simulink library "siltestlib"  (R2015b)
settings: Solver=VariableStepAuto  SolverMode=SingleTasking  StartTime=0.0  StopTime=10.0  RelTol=1e-3
settings Model: ExtModeArmWhenConnect=off  Creator=13188  LastModifiedBy=13188
settings DataIOCC: SaveFormat=Array  SignalLoggingSaveFormat=ModelDataLogs
settings OptimizationCC: BlockReduction=off  BooleanDataType=off
settings DebuggingCC: SaveWithParameterizedLinksMsg=none  UnderspecifiedInitializationDetection=Classic  MergeDetectMultiDrivingBlocksExec=none  SignalResolutionControl=TryResolveAllWithWarning  MultiTaskDSMMsg=warning  MultiTaskCondExecSysMsg=none  StrictBusMsg=None
settings HardwareCC: ProdBitPerPointer=32  ProdLargestAtomicFloat=None  ProdIntDivRoundTo=Undefined  ProdEndianess=Unspecified  ProdWordSize=32  ProdHWDeviceType=32-bit Generic  TargetUnknown=on
settings RTWCC: MakeCommand=make_rti  RetainRTWFile=on
settings ConfigComp: CovModelRefEnable=Off

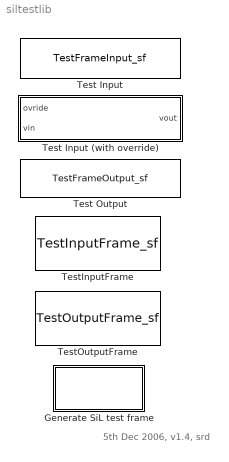
== system siltestlib ==
  note: 5th Dec 2006, v1.4, srd
  Generate SiL test frame : Subsystem  Description=Generate SiL\ntest frame  TreatAsAtomicUnit=on  mask(Generate SiL test frame button.){}
      mask help: Calls the function gen_sil_test_frame.
      settings: OpenFcn=|
      | if exist('gen_sil_test_frame','file'), gen_sil_test_frame(gcs); else,
      | fprintf('Error: gen_sil_test_frame is not on the matlab path.\n'); end
      mask Help: Calls the function gen_sil_test_frame.
      mask Display: fprintf('Generate SiL\ntest frame');
  Test Input : S-Function  FunctionName=TestFrameInput_sf  Parameters=varname,sampletime  SFunctionDeploymentMode=off  EnableBusSupport=off  mask(Test Input){varname=<UNDEFINED>, sampletime=-1}
      mask prompts: varname "Name:"; sampletime "Sample Time:"
      mask help: Outputs the value of a Test Input variable from an Excel spreadsheet when used with the runsiltest script. Otherwise outputs 0.
      mask Display: fprintf('Test Input:\n%s',varname);
  Test Input (with override) : Subsystem  mask(Test Input (with override)){varname=<UNDEFINED>, sampletime=-1}
      mask prompts: varname "Name:"; sampletime "Sample Time:"
      mask help: Outputs the input value if ovride >= 0.5 otherwise outputs the value from the SiLTest frame in the Matlab workspace. If not present then outputs 0.
      mask Help: Outputs the input value if ovride >= 0.5 otherwise outputs the value from the SiLTest frame in the Matlab workspace. If not present then outputs 0.
      mask Display:
      | fprintf('Test Input\n(with override):\n%s',varname);
      | port_label('input', 1, 'ovride')
      | port_label('input', 2, 'vin')
      | port_label('output', 1, 'vout')
  Test Output : S-Function  FunctionName=TestFrameOutput_sf  Parameters=varname,sampletime  SFunctionDeploymentMode=off  EnableBusSupport=off  mask(Test Output){varname=<UNDEFINED>, sampletime=-1}
      mask prompts: varname "Name:"; sampletime "Sample Time:"
      mask help: Samples the value of a Test Output variable from an Excel spreadsheet when used with the runsiltest script. Otherwise does nothing.
      mask Display: fprintf('Test Output:\n%s',varname);
  TestInputFrame : S-Function  FunctionName=TestInputFrame_sf  SFunctionDeploymentMode=off  EnableBusSupport=off  mask(TestInputFrame){}
      mask help:
      | Set the value of the obd array in Matlab from obdset input variables.
      | Update Matlab calibration from cal inputs.
      mask Help:
      | Set the value of the obd array in Matlab from obdset input variables.
      | Update Matlab calibration from cal inputs.
      mask Display: fprintf('TestInputFrame');
  TestOutputFrame : S-Function  FunctionName=TestOutputFrame_sf  SFunctionDeploymentMode=off  EnableBusSupport=off  mask(TestOutputFrame){}
      mask help: Sets the value of obdget output variables from the obd array in Matlab.
      mask Help: Sets the value of obdget output variables from the obd array in Matlab.
      mask Display: fprintf('TestOutputFrame');

== system siltestlib/Generate SiL test frame ==

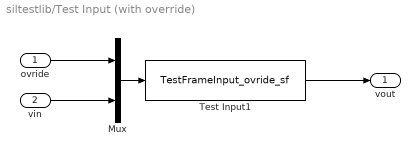
== system siltestlib/Test Input (with override) ==
  ovride : Inport
  vin : Inport  Port=2
  Mux : Mux  Inputs=2
  Test Input1 : S-Function  FunctionName=TestFrameInput_ovride_sf  Parameters=varname,sampletime  SFunctionDeploymentMode=off  EnableBusSupport=off
  vout : Outport
  wires:
  vin/1 -> Mux/2
  ovride/1 -> Mux/1
  Mux/1 -> Test Input1/1
  Test Input1/1 -> vout/1
